simulink model "generatorOfReferences"  (Simulink 8.3)
settings: Solver=FixedStepDiscrete  StartTime=0.0  StopTime=inf  FixedStep=Ts  RelTol=1e-3
InitFcn:
  | init_generatorOfReferences;
values from neighbouring files (symbols this model uses):
  directionOfOscillation = [0;1;0]    [init_generatorOfReferences.m]
  mask = zeros(ROBOT_DOF ,1)    [init_generatorOfReferences.m]
  noOscillationTime = 10    [init_generatorOfReferences.m]
  referenceParamsCoM = [0.03  0.05]    [init_generatorOfReferences.m]
  referenceParamsPost = [20*pi/180  0.05]    [init_generatorOfReferences.m]
undefined symbols (not defined in the file): localName, robotName, Ts
libraries: WBCLibrary x10
settings Model: Creator=daniele  LastModifiedBy=makaveli
settings DataIOCC: SignalLoggingSaveFormat=Dataset
settings OptimizationCC: ExpressionDepthLimit=2147483647
settings DebuggingCC: FcnCallInpInsideContextMsg=EnableAllAsWarning
settings SFSimCC: SimParseCustomCode=off

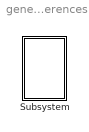
== system generatorOfReferences ==
  Subsystem : Subsystem  mask{robotName=robotName, Ts=Ts, localName=localName}
      mask prompts: robotName "robot name"; localName "module name"

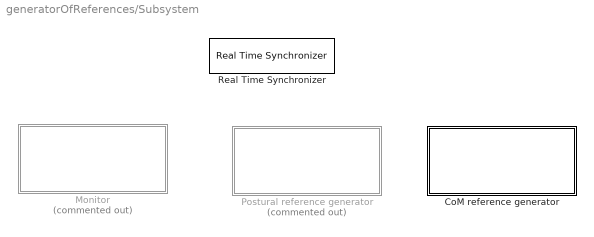
== system generatorOfReferences/Subsystem ==
  CoM reference generator : Subsystem
  Monitor : Subsystem  Commented=on
  Postural reference generator : Subsystem  Commented=on
  Real Time Synchronizer : WBCLibrary/Utilities/Real Time Synchronizer  Priority=-10  threadPeriod=Ts

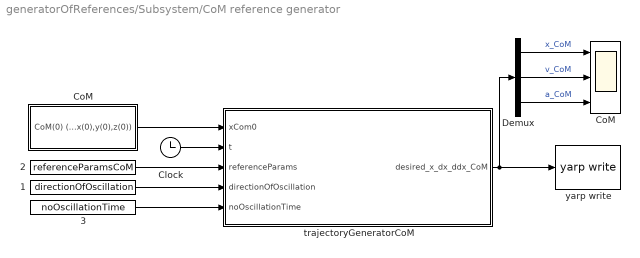
== system generatorOfReferences/Subsystem/CoM reference generator ==
  "    1" : Constant  Value=directionOfOscillation
  "    2" : Constant  Value=referenceParamsCoM
  "    3" : Constant  Value=noOscillationTime
  Clock : Clock
  CoM : Scope  NumInputPorts=3
      settings: ShowLegends=on  YMin=-5~-5~-5  YMax=5~5~5
  "CoM " : Subsystem
  Demux : Demux  Outputs=3
  trajectoryGeneratorCoM : MATLAB Function  TreatAsAtomicUnit=on
      settings: PermitHierarchicalResolution=ParametersOnly
  yarp write : WBCLibrary/Utilities/yarp write  port_name=outputPortCoM
  wires:
  "CoM "/1(CoM(0) (x(0),y(0),z(0))) -> trajectoryGeneratorCoM/1(xCom0)
  Clock/1 -> trajectoryGeneratorCoM/2(t)
  "    1"/1 -> trajectoryGeneratorCoM/4(directionOfOscillation)
  "    3"/1 -> trajectoryGeneratorCoM/5(noOscillationTime)
  trajectoryGeneratorCoM/1(desired_x_dx_ddx_CoM) -> yarp write/1, Demux/1
  Demux/3 -> CoM/3  "a_CoM"
  Demux/2 -> CoM/2  "v_CoM"
  Demux/1 -> CoM/1  "x_CoM"
  "    2"/1 -> trajectoryGeneratorCoM/3(referenceParams)

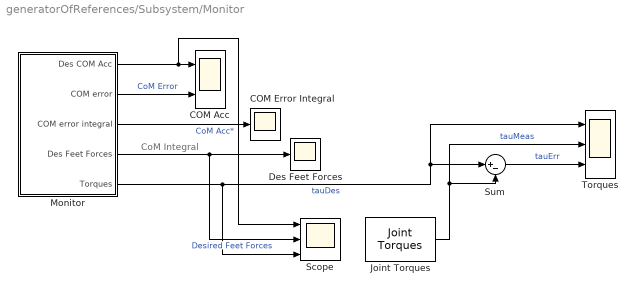
== system generatorOfReferences/Subsystem/Monitor ==
  note: CoM Integral
  COM Acc : Scope  NumInputPorts=2
      settings: ShowLegends=on  YMin=-0.4~-0.02  YMax=0.2~0.04  SaveName=ScopeData5
  COM Error Integral : Scope
      settings: YMin=-0.7  YMax=0.1  SaveName=ScopeData4
  Des Feet Forces : Scope
      settings: TimeRange=10  YMin=-10  YMax=120  SaveName=ScopeData2
  Joint Torques : WBCLibrary/wholeBodyStates/Joint Torques  robotName=robotName  localName=localName
  Monitor : Subsystem
  Scope : Scope  NumInputPorts=3
      settings: ShowLegends=on  YMin=-0.4~-20~-20  YMax=0.3~160~10
  Sum : Sum  Inputs=|+-
  Torques : Scope  NumInputPorts=3
      settings: YMin=-1~-5~-5  YMax=1~5~5  SaveName=ScopeData3
  wires:
  Monitor/1(Des COM Acc) -> Scope/1, COM Acc/1  "CoM Acc*"
  Monitor/4(Des Feet Forces) -> Scope/2, Des Feet Forces/1  "Desired Feet Forces"
  Monitor/5(Torques) -> Scope/3, Sum/1, Torques/1  "tauDes"
  Monitor/2(COM error) -> COM Acc/2  "CoM Error"
  Monitor/3(COM error integral) -> COM Error Integral/1
  Joint Torques/1 -> Sum/2, Torques/2  "tauMeas"
  Sum/1 -> Torques/3  "tauErr"

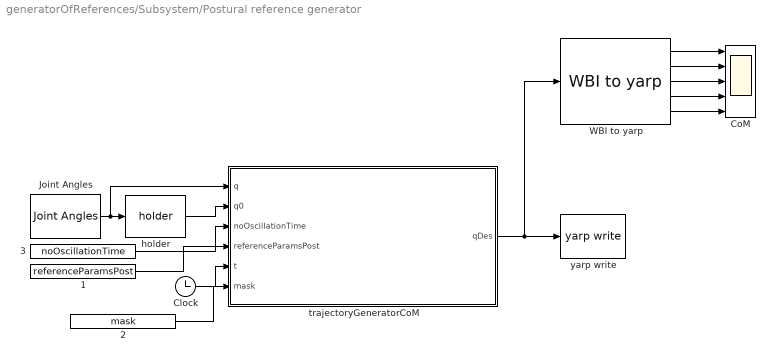
== system generatorOfReferences/Subsystem/Postural reference generator ==
  "    1" : Constant  Value=referenceParamsPost
  "    2" : Constant  Value=mask
  "    3" : Constant  Value=noOscillationTime
  Clock : Clock
  CoM : Scope  NumInputPorts=5
      settings: ShowLegends=on  YMin=-5~-5~-5~-5~-5  YMax=5~5~5~5~5
  Joint Angles : WBCLibrary/wholeBodyStates/Joint Angles  robotName=robotName  localName=localName
  WBI to yarp : WBCLibrary/Utilities/WBI to yarp
  "holder " : WBCLibrary/Utilities/holder 
  trajectoryGeneratorCoM : MATLAB Function  TreatAsAtomicUnit=on
      settings: PermitHierarchicalResolution=ParametersOnly
  yarp write : WBCLibrary/Utilities/yarp write  port_name=outputPortPostural
  wires:
  trajectoryGeneratorCoM/1(qDes) -> WBI to yarp/1, yarp write/1
  Joint Angles/1 -> trajectoryGeneratorCoM/1(q), "holder "/1
  "    3"/1 -> trajectoryGeneratorCoM/3(noOscillationTime)
  Clock/1 -> trajectoryGeneratorCoM/5(t)
  "holder "/1 -> trajectoryGeneratorCoM/2(q0)
  "    1"/1 -> trajectoryGeneratorCoM/4(referenceParamsPost)
  "    2"/1 -> trajectoryGeneratorCoM/6(mask)
  WBI to yarp/3 -> CoM/3
  WBI to yarp/2 -> CoM/2
  WBI to yarp/1 -> CoM/1
  WBI to yarp/4 -> CoM/4
  WBI to yarp/5 -> CoM/5

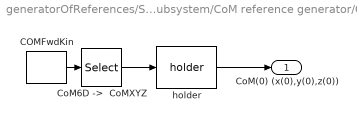
== system generatorOfReferences/Subsystem/CoM reference generator/CoM  ==
  "COMFwdKin " : WBCLibrary/wholeBodyModel/Forward Kinematics/COMFwdKin   robotName=robotName  localName=localName
  "CoM6D ->  CoMXYZ" : Selector  InputPortWidth=7  Indices=[1 2 3]
  "holder " : WBCLibrary/Utilities/holder 
  CoM(0) (x(0),y(0),z(0)) : Outport
  wires:
  "COMFwdKin "/1 -> "CoM6D ->  CoMXYZ"/1
  "CoM6D ->  CoMXYZ"/1 -> "holder "/1
  "holder "/1 -> CoM(0) (x(0),y(0),z(0))/1

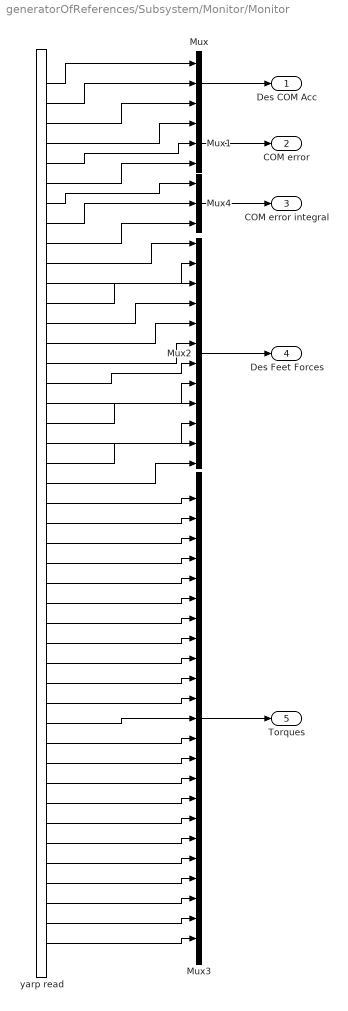
== system generatorOfReferences/Subsystem/Monitor/Monitor ==
  Mux : Mux  Inputs=3
  Mux1 : Mux  Inputs=3
  Mux2 : Mux  Inputs=12
  Mux3 : Mux  Inputs=23
  Mux4 : Mux  Inputs=3
  yarp read : WBCLibrary/Utilities/yarp read  from=['/torqueBalancing/monitor:o']  to='...'  num=44  blocking=off  timestamp=off  autoconnect=on
  Des COM Acc : Outport
  COM error : Outport  Port=2
  COM error integral : Outport  Port=3
  Des Feet Forces : Outport  Port=4
  Torques : Outport  Port=5
  wires:
  Mux/1 -> Des COM Acc/1
  Mux2/1 -> Des Feet Forces/1
  Mux1/1 -> COM error/1
  Mux3/1 -> Torques/1
  Mux4/1 -> COM error integral/1
  yarp read/3 -> Mux/3
  yarp read/2 -> Mux/2
  yarp read/1 -> Mux/1
  yarp read/6 -> Mux1/3
  yarp read/4 -> Mux1/1
  yarp read/5 -> Mux1/2
  yarp read/9 -> Mux4/3
  yarp read/8 -> Mux4/2
  yarp read/7 -> Mux4/1
  yarp read/19 -> Mux2/10
  yarp read/11 -> Mux2/2
  yarp read/20 -> Mux2/11
  yarp read/17 -> Mux2/8
  yarp read/18 -> Mux2/9
  yarp read/12 -> Mux2/3
  yarp read/14 -> Mux2/5
  yarp read/15 -> Mux2/6
  yarp read/13 -> Mux2/4
  yarp read/10 -> Mux2/1
  yarp read/21 -> Mux2/12
  yarp read/16 -> Mux2/7
  yarp read/25 -> Mux3/4
  yarp read/24 -> Mux3/3
  yarp read/39 -> Mux3/18
  yarp read/38 -> Mux3/17
  yarp read/28 -> Mux3/7
  yarp read/43 -> Mux3/22
  yarp read/37 -> Mux3/16
  yarp read/22 -> Mux3/1
  yarp read/23 -> Mux3/2
  yarp read/40 -> Mux3/19
  yarp read/34 -> Mux3/13
  yarp read/35 -> Mux3/14
  yarp read/30 -> Mux3/9
  yarp read/41 -> Mux3/20
  yarp read/29 -> Mux3/8
  yarp read/42 -> Mux3/21
  yarp read/27 -> Mux3/6
  yarp read/32 -> Mux3/11
  yarp read/31 -> Mux3/10
  yarp read/26 -> Mux3/5
  yarp read/36 -> Mux3/15
  yarp read/33 -> Mux3/12
  yarp read/44 -> Mux3/23

== matlab function Subsystem/CoM reference generator/trajectoryGeneratorCoM ==
  data: desired_x_dx_ddx_CoM output double; xCom0 input double; t input double; referenceParams input double; directionOfOscillation input double; noOscillationTime input double
function desired_x_dx_ddx_CoM = fcn(xCom0,t,referenceParams,directionOfOscillation,noOscillationTime)
%#codegen


if t > noOscillationTime
    A = referenceParams(1);
else
    A = 0;
end
f = referenceParams(2);

xcomDes    = xCom0 + A*sin(2*pi*f*t)*directionOfOscillation;
% xcomDes(1) =  xcomDes(1) + 0.01;
xDcomDes   =         A*2*pi*f*cos(2*pi*f*t)*directionOfOscillation;
xDDcomDes  =        -A*(2*pi*f)^2*sin(2*pi*f*t)*directionOfOscillation;

desired_x_dx_ddx_CoM = [xcomDes;xDcomDes;xDDcomDes];

== matlab function Subsystem/Postural reference generator/trajectoryGeneratorCoM ==
  data: qDes output double; q input double; q0 input double; noOscillationTime input double; referenceParamsPost input double; t input double; mask input double
function qDes = fcn(q,q0,noOscillationTime,referenceParamsPost,t,mask)
%#codegen

qDes = q0;
if t > noOscillationTime
    qDes = q0 + referenceParamsPost(1)*sin(referenceParamsPost(2)*(t-noOscillationTime)).*mask;
end
